simulink model "intro"  (R2020b)
settings: Solver=VariableStepAuto  StartTime=0.0  StopTime=10.0  RelTol=1e-3
settings Model: Creator=dongwei  LastModifiedBy=dongwei

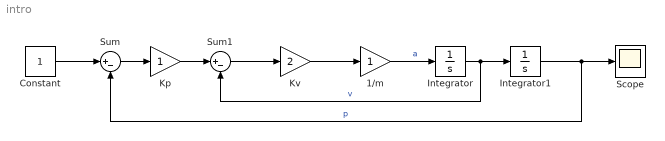
== system intro ==
  1/m : Gain
  Constant : Constant
  Integrator : Integrator
  Integrator1 : Integrator
  Kp : Gain
  Kv : Gain  Gain=2
  Scope : Scope
  Sum : Sum  Inputs=|+-
  Sum1 : Sum  Inputs=|+-
  wires:
  Integrator/1 -> Sum1/2, Integrator1/1  "v"
  Integrator1/1 -> Sum/2, Scope/1  "p"
  1/m/1 -> Integrator/1  "a"
  Sum/1 -> Kp/1
  Constant/1 -> Sum/1
  Kp/1 -> Sum1/1
  Kv/1 -> 1/m/1
  Sum1/1 -> Kv/1
